simulink model "MDS_simulink"  (R2020b)
settings: Solver=VariableStepAuto  StartTime=0.0  StopTime=20  RelTol=1e-3
settings Model: Creator=Admin  LastModifiedBy=Admin

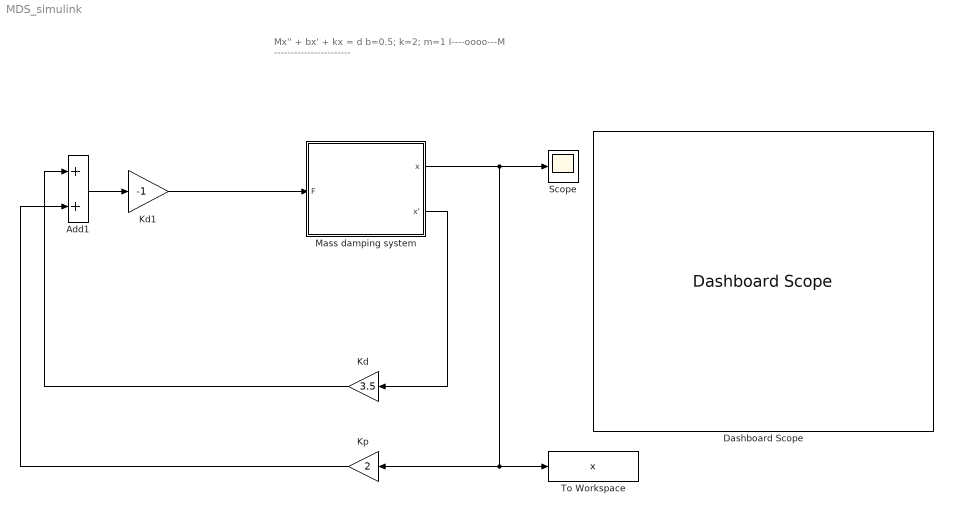
== system MDS_simulink ==
  note: Mx'' + bx' + kx = d
      | b=0.5; k=2; m=1
      |
      | I----oooo---M
      | -----------------------
  Add1 : Sum
  Dashboard Scope : DashboardScope
  Kd : Gain  Gain=3.5
  Kd1 : Gain  Gain=-1
  Kp : Gain  Gain=2
  Mass damping system : Subsystem
  Scope : Scope
  To Workspace : ToWorkspace  VariableName=x  SampleTime=-1
  wires:
  Add1/1 -> Kd1/1
  Kd/1 -> Add1/1
  Kp/1 -> Add1/2
  Mass damping system/1(x) -> To Workspace/1, Kp/1, Scope/1
  Kd1/1 -> Mass damping system/1(F)
  Mass damping system/2(x') -> Kd/1

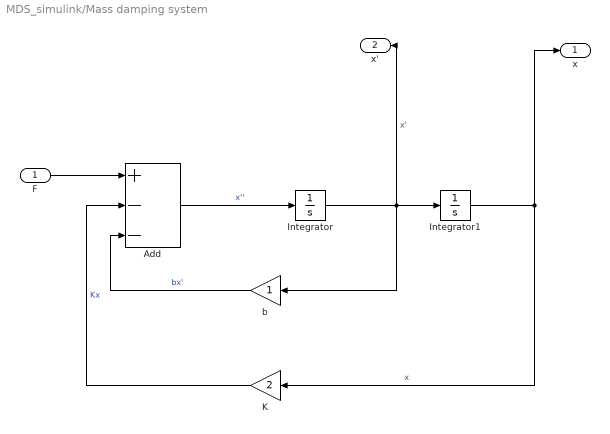
== system MDS_simulink/Mass damping system ==
  F : Inport
  Add : Sum  Inputs=+--
  Integrator : Integrator
  Integrator1 : Integrator  InitialCondition=1
  K : Gain  Gain=2
  b : Gain
  x : Outport
  x' : Outport  Port=2
  wires:
  Add/1 -> Integrator/1  "x''"
  Integrator1/1 -> x/1, K/1  "x"
  Integrator/1 -> x'/1, b/1, Integrator1/1  "x'"
  b/1 -> Add/3  "bx'"
  K/1 -> Add/2  "Kx"
  F/1 -> Add/1
